simulink model "do178b_dhc2_rev_new"  (R2021b)
settings: Solver=ode23  StartTime=0.0  StopTime=25  MaxStep=1/40  RelTol=1e-2  AbsTol=1e-3  EnableMultiTasking=on
PreLoadFcn:
  | load asbdhc2_init;
  | Autopilot_bus;
model workspace (MAT data in the model file):
  ALT_Mode = [0 0 0 0 0 0 0 0 0 0 0 0 ... (1001 elements, 1001x1)]
  ALT_Ref = [991.703720962 991.703720962 991.703720962 991.703720962 991.703720962 991.703720962 991.703720962 991.703720962 991.703720962 991.703720962 991.703720962 991.703720962 ... (1001 elements, 1001x1)]
  AP_Eng = [1 1 1 1 1 1 1 1 1 1 1 1 ... (1001 elements, 1001x1)]
  AilCmdv = [0; 0; 0]
  Ail_cmd : timeseries (value not decoded)
  FR = [0; 0]
  Ft = [0 0.333333333333 0.333333333333 0.333333333333 0.333333333333 0.333333333333 0.333333333333 0.333333333333 0.333333333333 0.333333333333 0.333333333333 0.333333333333 ... (1001 elements, 1001x1)]
  HDG_Mode = [0 0 0 0 0 0 0 0 0 0 0 0 ... (1001 elements, 1001x1)]
  HDG_Ref = [29.7066688805 29.7066688805 29.7066688805 29.7066688805 29.7066688805 29.7066688805 29.7066688805 29.7066688805 29.7066688805 29.7066688805 29.7066688805 29.7066688805 ... (1001 elements, 1001x1)]
  InputSize = 2
  N = 37
  PhiRefv = [0; 0; 0]
  Phi_Ref : timeseries (value not decoded)
  Phiv = [0; 0; 0]
  Pwheel = [2.59796598511 2.59796598511 2.59796598511 2.59796598511 2.59796598511 2.59796598511 2.59796598511 2.59796598511 2.59796598511 2.59796598511 2.59796598511 2.59796598511 ... (1001 elements, 1001x1)]
  Roll_Mode = [1 1 1 1 1 1 1 1 1 1 1 1 ... (1001 elements, 1001x1)]
  TimeSteps = 1001
  Tkv = [0; 0; 0]
  TurnK = [-15.9132354515 -15.9132354515 -15.9132354515 -15.9132354515 -15.9132354515 -15.9132354515 -15.9132354515 -15.9132354515 -15.9132354515 -15.9132354515 -15.9132354515 -15.9132354515 ... (1001 elements, 1001x1)]
  X = [1 1 1 0 0 0 0 0 1 81.536789931 -1.01532751936 38.5971284353 ... (24 elements, 1x24)]
  a = 0.726747501556
  a1 = [0.30275909672 0.30275909672 0.30275909672 0.30275909672 0.30275909672 0.30275909672 0.30275909672 0.30275909672 0.30275909672 0.30275909672 0.30275909672 0.30275909672 ... (1001 elements, 1x1001)]
  apin : object (value not decoded)
  apsin : time (value not decoded)
  curPath = 'C:\Python-Workspace\thesis\new FSE2019\ModeTestingData\Problems'
  d = 25
  hws : Simulink.ModelWorkspace (value not decoded)
  i = 9
  inertial : object (value not decoded)
  j = 8
  list : object (value not decoded)
  modelpath = 'C:\Python-Workspace\thesis\new FSE2019\Benchmark\Simulink Models\autopilot\aprevised\'
  models : object (value not decoded)
  n = 1
  nbrInputs = 8
  req = 'R12.1'
  rollOut = []
  simOut : Simulink.SimulationOutput (value not decoded)
  t = [0 0.025 0.05 0.075 0.1 0.125 0.15 0.175 0.2 0.225 0.25 0.275 ... (1001 elements, 1x1001)]
undefined symbols (not defined in the file): beaver_b, beaver_c, beaver_init_p, beaver_init_pitch, beaver_init_q, beaver_init_r, beaver_init_roll, beaver_mass, Cl0, Cl_alpha2_dpt, Cl_beta, Cl_da, Cl_da_alpha, Cl_dr, Cl_p, Cl_r, Cm0, Cm_alpha, Cm_alpha2, Cm_beta2, Cm_de, Cm_df, Cm_dpt, Cm_q, Cm_r, Cn0, Cn_beta, Cn_beta3, Cn_da, Cn_dpt3, Cn_dr, Cn_p, Cn_q, Cn_r, Cx0, Cx_alpha, Cx_alpha2, Cx_alpha3, Cx_df, Cx_df_alpha, Cx_dpt, Cx_dpt2_alpha, Cx_dr, Cx_q, Cy0, Cy_beta, Cy_da, Cy_dr, Cy_dr_alpha, Cy_p, Cy_r, Cz0, Cz_alpha, Cz_alpha3, Cz_de, Cz_de_beta, Cz_df, Cz_df_alpha, Cz_dpt, Cz_q ... (+9)
libraries: aerolibconvert2 x6, simulink x6, aerolibobsolete x5, aerolibasang x3, aerolibwind2 x3, aerolibadyn x1, aerolibatmos2 x1
(part 3 of 3)

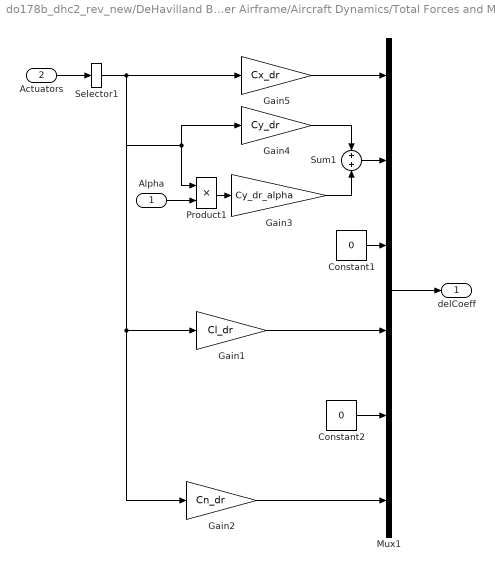
== system do178b_dhc2_rev_new/DeHavilland Beaver Airframe/Aircraft Dynamics/Total Forces and Moments/Aerodynamics/Actuator Increments/Rudder ==
  Alpha : Inport
  Actuators : Inport  Port=2
  Constant1 : Constant  Value=0
  Constant2 : Constant  Value=0
  Gain1 : Gain  Gain=Cl_dr  SaturateOnIntegerOverflow=on  OutDataTypeStr=Inherit: Same as input  ParamDataTypeStr=Inherit: Same as input
  Gain2 : Gain  Gain=Cn_dr  SaturateOnIntegerOverflow=on  OutDataTypeStr=Inherit: Same as input  ParamDataTypeStr=Inherit: Same as input
  Gain3 : Gain  Gain=Cy_dr_alpha  SaturateOnIntegerOverflow=on  OutDataTypeStr=Inherit: Same as input  ParamDataTypeStr=Inherit: Same as input
  Gain4 : Gain  Gain=Cy_dr  SaturateOnIntegerOverflow=on  OutDataTypeStr=Inherit: Same as input  ParamDataTypeStr=Inherit: Same as input
  Gain5 : Gain  Gain=Cx_dr  SaturateOnIntegerOverflow=on  OutDataTypeStr=Inherit: Same as input  ParamDataTypeStr=Inherit: Same as input
  Mux1 : Mux  Inputs=6
  Product1 : Product  InputSameDT=on  SaturateOnIntegerOverflow=on  OutDataTypeStr=Inherit: Same as first input
  Selector1 : Selector  InputPortWidth=4  IndexOptions=Index vector (dialog)  Indices=3  OutputSizes=1
  Sum1 : Sum  SaturateOnIntegerOverflow=on
  delCoeff : Outport  VectorParamsAs1DForOutWhenUnconnected=off
  wires:
  Gain5/1 -> Mux1/1
  Gain4/1 -> Sum1/1
  Gain3/1 -> Sum1/2
  Gain1/1 -> Mux1/4
  Gain2/1 -> Mux1/6
  Product1/1 -> Gain3/1
  Alpha/1 -> Product1/2
  Mux1/1 -> delCoeff/1
  Actuators/1 -> Selector1/1
  Sum1/1 -> Mux1/2
  Constant1/1 -> Mux1/3
  Constant2/1 -> Mux1/5
  Selector1/1 -> Gain5/1, Gain4/1, Gain1/1, Gain2/1, Product1/1

== system do178b_dhc2_rev_new/DeHavilland Beaver Airframe/Aircraft Dynamics/Total Forces and Moments/Aerodynamics/Body Rate Damping/p ==
  Constant1 : Constant  Value=0
  Constant2 : Constant  Value=Cy_p
  Constant3 : Constant  Value=Cl_p
  Constant4 : Constant  Value=Cn_p
  Mux1 : Mux  Inputs=6
  delCoeff : Outport  VectorParamsAs1DForOutWhenUnconnected=off
  wires:
  Constant2/1 -> Mux1/2
  Mux1/1 -> delCoeff/1
  Constant1/1 -> Mux1/5, Mux1/3, Mux1/1
  Constant4/1 -> Mux1/6
  Constant3/1 -> Mux1/4

== system do178b_dhc2_rev_new/DeHavilland Beaver Airframe/Aircraft Dynamics/Total Forces and Moments/Aerodynamics/Body Rate Damping/q ==
  Constant1 : Constant  Value=0
  Constant2 : Constant  Value=Cz_q
  Constant3 : Constant  Value=Cx_q
  Constant4 : Constant  Value=Cm_q
  Constant5 : Constant  Value=Cn_q
  Mux1 : Mux  Inputs=6
  delCoeff : Outport  VectorParamsAs1DForOutWhenUnconnected=off
  wires:
  Constant2/1 -> Mux1/3
  Constant5/1 -> Mux1/6
  Constant1/1 -> Mux1/4, Mux1/2
  Constant4/1 -> Mux1/5
  Constant3/1 -> Mux1/1
  Mux1/1 -> delCoeff/1

== system do178b_dhc2_rev_new/DeHavilland Beaver Airframe/Aircraft Dynamics/Total Forces and Moments/Aerodynamics/Body Rate Damping/r ==
  Constant : Constant  Value=0
  Constant1 : Constant  Value=Cy_r
  Constant2 : Constant  Value=Cl_r
  Constant3 : Constant  Value=Cm_r
  Constant4 : Constant  Value=Cn_r
  Mux1 : Mux  Inputs=6
  delCoeff : Outport  VectorParamsAs1DForOutWhenUnconnected=off
  wires:
  Constant3/1 -> Mux1/5
  Constant1/1 -> Mux1/2
  Constant4/1 -> Mux1/6
  Constant2/1 -> Mux1/4
  Constant/1 -> Mux1/3, Mux1/1
  Mux1/1 -> delCoeff/1
